simulink model "Grading"  (R2018b)
settings: Solver=FixedStepDiscrete  StartTime=0.0  StopTime=10.0  RelTol=1e-3
settings Model: Creator=karim  LastModifiedBy=karim
settings OptimizationCC: DefaultParameterBehavior=Inlined  EnhancedBackFolding=on  PassReuseOutputArgsAs=Individual arguments  OptimizeBlockOrder=speed  DifferentSizesBufferReuse=on  OptimizationCustomize=off
settings DebuggingCC: UnderspecifiedInitializationDetection=Classic  MergeDetectMultiDrivingBlocksExec=none  ParameterTunabilityLossMsg=error
settings ModelReferenceCC: PropagateSignalLabelsOutOfModel=off
settings SFSimCC: MATLABDynamicMemAlloc=off
settings RTWCC: SystemTargetFile=ert.tlc  GenCodeOnly=on  TemplateMakefile=ert_default_tmf  GenerateReport=on  IncludeHyperlinkInReport=on  LaunchReport=on  GenerateTraceInfo=on  GenerateTraceReport=on  GenerateTraceReportSl=on  GenerateTraceReportSf=on  GenerateTraceReportEml=on
settings CodeAppCC: ForceParamTrailComments=on  IgnoreCustomStorageClasses=off  OperatorAnnotations=on  SimulinkDataObjDesc=on  SFDataObjDesc=on  InsertBlockDesc=on
settings ERTTargetCC: TargetLangStandard=C99 (ISO)  GenerateSampleERTMain=on  InlinedParameterPlacement=NonHierarchical  ERTCustomFileTemplate=example_file_process.tlc

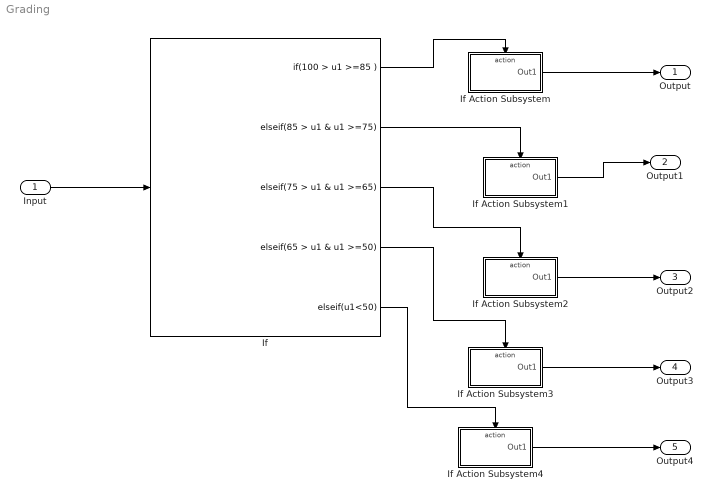
== system Grading ==
  Input : Inport
  If : If  IfExpression=100 > u1 >=85  ElseIfExpressions=85 > u1 & u1 >=75 , 75 > u1 & u1 >=65 , 65 > u1 & u1 >=50 , u1<50  ShowElse=off
  If Action Subsystem : Subsystem  TreatAsAtomicUnit=on
  If Action Subsystem1 : Subsystem  TreatAsAtomicUnit=on
  If Action Subsystem2 : Subsystem  TreatAsAtomicUnit=on
  If Action Subsystem3 : Subsystem  TreatAsAtomicUnit=on
  If Action Subsystem4 : Subsystem  TreatAsAtomicUnit=on
  Output : Outport
  Output1 : Outport  Port=2
  Output2 : Outport  Port=3
  Output3 : Outport  Port=4
  Output4 : Outport  Port=5
  wires:
  If/1 -> If Action Subsystem/Action
  If/2 -> If Action Subsystem1/Action
  If/3 -> If Action Subsystem2/Action
  If/4 -> If Action Subsystem3/Action
  If/5 -> If Action Subsystem4/Action
  Input/1 -> If/1
  If Action Subsystem/1(Out1) -> Output/1
  If Action Subsystem1/1(Out1) -> Output1/1
  If Action Subsystem2/1(Out1) -> Output2/1
  If Action Subsystem3/1(Out1) -> Output3/1
  If Action Subsystem4/1(Out1) -> Output4/1

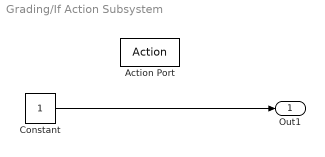
== system Grading/If Action Subsystem ==
  Action Port : ActionPort  ActionType=then
  Constant : Constant
  Out1 : Outport
  wires:
  Constant/1 -> Out1/1

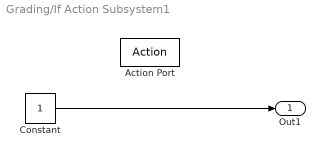
== system Grading/If Action Subsystem1 ==
  Action Port : ActionPort  ActionType=elseif
  Constant : Constant
  Out1 : Outport
  wires:
  Constant/1 -> Out1/1

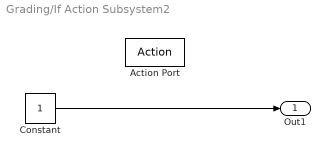
== system Grading/If Action Subsystem2 ==
  Action Port : ActionPort  ActionType=elseif
  Constant : Constant
  Out1 : Outport
  wires:
  Constant/1 -> Out1/1

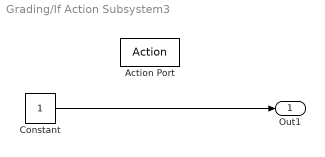
== system Grading/If Action Subsystem3 ==
  Action Port : ActionPort  ActionType=elseif
  Constant : Constant
  Out1 : Outport
  wires:
  Constant/1 -> Out1/1

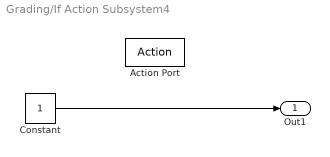
== system Grading/If Action Subsystem4 ==
  Action Port : ActionPort  ActionType=elseif
  Constant : Constant
  Out1 : Outport
  wires:
  Constant/1 -> Out1/1
